simulink model "Simulink_simulation2"  (R2014a)
settings: Solver=ode15s  StartTime=0.0  StopTime=100  RelTol=1e-3
libraries: vrlib x1
settings Model: Creator=xp  LastModifiedBy=xp

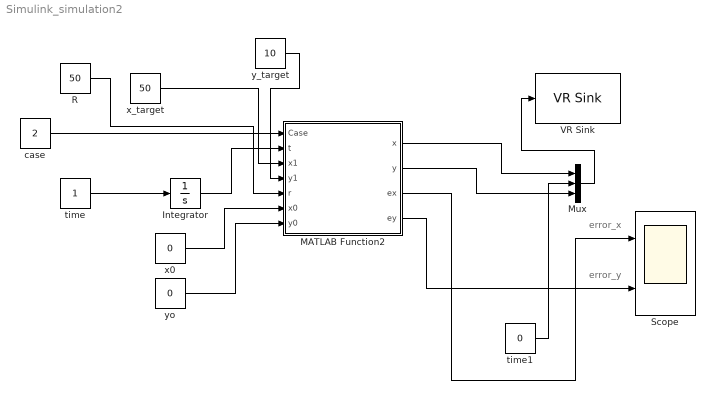
== system Simulink_simulation2 ==
  note: error_y
  note: error_x
  Integrator : Integrator
  MATLAB Function2 : MATLAB Function  TreatAsAtomicUnit=on
  Mux : Mux  Inputs=3
  R : Constant  Value=50
  Scope : Scope  NumInputPorts=2
      settings: YMin=-5~-5  YMax=5~5
  VR Sink : vrlib/VR Sink  InstantiateOnLoad=on  SampleTime=1  ViewEnable=on  RemoteChange=off  RemoteView=off  FieldsWritten=ball.translation.3.1.1.double  WorldFileName=Ball_Plate.wrl  AutoView=off  VideoDimensions=[]  AllowVariableSize=off
  case : Constant  Value=2
  time : Constant
  time1 : Constant  Value=0
  x0 : Constant  Value=0
  x_target : Constant  Value=50
  y_target : Constant  Value=10
  yo : Constant  Value=0
  wires:
  x_target/1 -> MATLAB Function2/3(x1)
  y_target/1 -> MATLAB Function2/4(y1)
  MATLAB Function2/1(x) -> Mux/1
  time/1 -> Integrator/1
  Integrator/1 -> MATLAB Function2/2(t)
  Mux/1 -> VR Sink/1
  time1/1 -> Mux/2
  R/1 -> MATLAB Function2/5(r)
  x0/1 -> MATLAB Function2/6(x0)
  yo/1 -> MATLAB Function2/7(y0)
  case/1 -> MATLAB Function2/1(Case)
  MATLAB Function2/3(ex) -> Scope/1
  MATLAB Function2/4(ey) -> Scope/2
  MATLAB Function2/2(y) -> Mux/3

== matlab function Simulink_simulation2/MATLAB Function2 ==
  data: Case input; t input; x1 input; x output; y1 input; r input; x0 input; y0 input; y output; ex output; ey output
function [x,y,ex,ey] = fcn( Case ,t, x1, y1, r, x0, y0)
t = linspace(0,t,1);
kx1 = (81243429*x1)/81250000 + (45737168756571*x1.*exp(-325000.*t))/(17164062500000000000*x1 - 52812500000000*(2*x1)^(1/2) + 81250000) - (exp(-t./(2*x1)^(1/2)).*(281460000*x1^2 - 81243429*(2*x1)^(5/2) + 105616457700000*x1^3))/(500*x1*(211250000000*x1 - 650000*(2*x1)^(1/2) + 1)) - (t.*exp(-t./(2*x1)^(1/2))*(81243429*(2*x1)^(5/2) - 91474987460574*x1^2*(2*x1)^(1/2) + 281460000*x1^2 + 105616457700000*x1^3))/(500*x1*(2*x1)^(1/2)*(211250000000*x1 - 650000*(2*x1)^(1/2) + 1));
ky1 = (81243429*y1)/81250000 + (45737168756571*y1.*exp(-325000.*t))/(17164062500000000000*y1 - 52812500000000*(2*y1)^(1/2) + 81250000) - (exp(-t./(2*y1)^(1/2)).*(281460000*y1^2 - 81243429*(2*y1)^(5/2) + 105616457700000*y1^3))/(500*y1*(211250000000*y1 - 650000*(2*y1)^(1/2) + 1)) - (t.*exp(-t./(2*y1)^(1/2))*(81243429*(2*y1)^(5/2) - 91474987460574*y1^2*(2*y1)^(1/2) + 281460000*y1^2 + 105616457700000*y1^3))/(500*y1*(2*y1)^(1/2)*(211250000000*y1 - 650000*(2*y1)^(1/2) + 1));
kx2 = kx1(1,1);
ky2 = ky1(1,1);
switch(Case)
    case 1
       ex = x1-kx2;
       ey = y1-ky2;
    case 2
        
        if t>60
            
        x1 = r*cosd(t-15);
        y1 = r*sind(t-15);
        
kx1 = (81243429*x1)/81250000 + (45737168756571*x1.*exp(-325000.*t))/(17164062500000000000*x1 - 52812500000000*(norm(2*x1))^(1/2) + 81250000) - (exp(-t./(norm(2*x1))^(1/2)).*(281460000*x1^2 - 81243429*(norm(2*x1))^(5/2) + 105616457700000*x1^3))/(500*x1*(211250000000*x1 - 650000*(norm(2*x1))^(1/2) + 1)) - (t.*exp(-t./(norm(2*x1))^(1/2))*(81243429*(norm(2*x1))^(5/2) - 91474987460574*x1^2*(norm(2*x1))^(1/2) + 281460000*x1^2 + 105616457700000*x1^3))/(500*x1*(norm(2*x1))^(1/2)*(211250000000*x1 - 650000*(norm(2*x1))^(1/2) + 1));
ky1 = (81243429*y1)/81250000 + (45737168756571*y1.*exp(-325000.*t))/(17164062500000000000*y1 - 52812500000000*(norm(2*y1))^(1/2) + 81250000) - (exp(-t./(norm(2*y1))^(1/2)).*(281460000*y1^2 - 81243429*(norm(2*y1))^(5/2) + 105616457700000*y1^3))/(500*y1*(211250000000*y1 - 650000*(norm(2*y1))^(1/2) + 1)) - (t.*exp(-t./(norm(2*y1))^(1/2))*(81243429*(norm(2*y1))^(5/2) - 91474987460574*y1^2*(norm(2*y1))^(1/2) + 281460000*y1^2 + 105616457700000*y1^3))/(500*y1*(norm(2*y1))^(1/2)*(211250000000*y1 - 650000*(norm(2*y1))^(1/2) + 1));
kx2 = kx1(1,1);
ky2 = ky1(1,1);
        else
            x1 = r*cosd(45);
        y1 = r*sind(45);
kx1 = (81243429*x1)/81250000 + (45737168756571*x1.*exp(-325000.*t))/(17164062500000000000*x1 - 52812500000000*(norm(2*x1))^(1/2) + 81250000) - (exp(-t./(norm(2*x1))^(1/2)).*(281460000*x1^2 - 81243429*(norm(2*x1))^(5/2) + 105616457700000*x1^3))/(500*x1*(211250000000*x1 - 650000*(norm(2*x1))^(1/2) + 1)) - (t.*exp(-t./(norm(2*x1))^(1/2))*(81243429*(norm(2*x1))^(5/2) - 91474987460574*x1^2*(norm(2*x1))^(1/2) + 281460000*x1^2 + 105616457700000*x1^3))/(500*x1*(norm(2*x1))^(1/2)*(211250000000*x1 - 650000*(norm(2*x1))^(1/2) + 1));
kx2 = kx1(1,1);
ky1 = (81243429*y1)/81250000 + (45737168756571*y1.*exp(-325000.*t))/(17164062500000000000*y1 - 52812500000000*(norm(2*y1))^(1/2) + 81250000) - (exp(-t./(norm(2*y1))^(1/2)).*(281460000*y1^2 - 81243429*(norm(2*y1))^(5/2) + 105616457700000*y1^3))/(500*y1*(211250000000*y1 - 650000*(norm(2*y1))^(1/2) + 1)) - (t.*exp(-t./(norm(2*y1))^(1/2))*(81243429*(norm(2*y1))^(5/2) - 91474987460574*y1^2*(norm(2*y1))^(1/2) + 281460000*y1^2 + 105616457700000*y1^3))/(500*y1*(norm(2*y1))^(1/2)*(211250000000*y1 - 650000*(norm(2*y1))^(1/2) + 1));
ky2 = ky1(1,1);

            
        end
        
       
       end

x = kx2;
y = ky2;
 ex = x1-kx2;
       ey = y1-ky2;
